simulink model "udp_simulink_example"  (R2022b)
settings: Solver=VariableStepAuto  StartTime=0.0  StopTime=10.0  RelTol=1e-3
libraries: dspnetwork x2
settings Model: Creator=emu  LastModifiedBy=emu

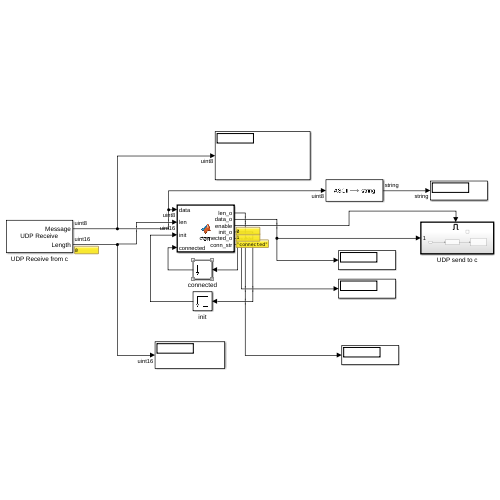
[thumbnail: Simulink's stored preview of the top-level diagram]
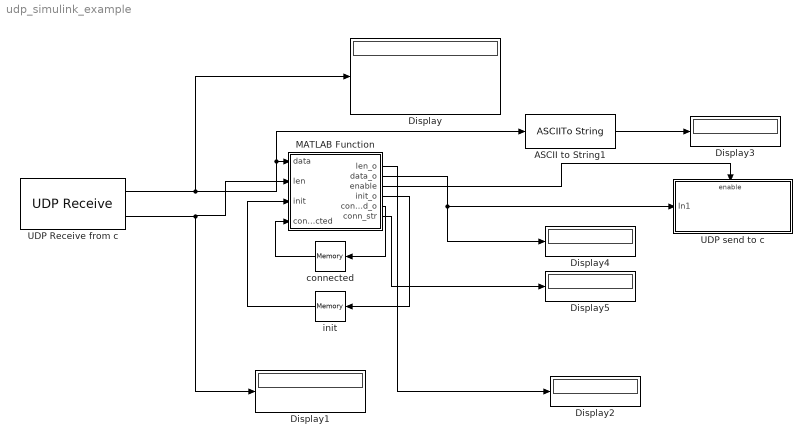
== system udp_simulink_example ==
  ASCII to String1 : ASCIIToString
  Display{,1..5} (6 alike) : Display
  MATLAB Function : MATLAB Function  TreatAsAtomicUnit=on
  UDP Receive from c : dspnetwork/UDP Receive  localURL='0.0.0.0'  localPort=8080  remoteURL='127.0.0.1'  remotePort=-1  recvBufferSize=1024  dims=1024  signalDatatype=uint8  isComplex=off  isVarSize=off  showBlockingTime=off  blockingTime=0  sampletime=1  blockPlatform=[]
      settings: LibrarySourceBlock=dspsrcs4/UDP Receive
  UDP send to c : Subsystem
  connected : Memory
  init : Memory
  wires:
  UDP Receive from c/1 -> ASCII to String1/1, MATLAB Function/1(data), Display/1
  UDP Receive from c/2 -> Display1/1, MATLAB Function/2(len)
  MATLAB Function/1(len_o) -> Display2/1
  connected/1 -> MATLAB Function/4(connected)
  ASCII to String1/1 -> Display3/1
  MATLAB Function/2(data_o) -> Display4/1, UDP send to c/1(In1)
  MATLAB Function/3(enable) -> UDP send to c/Enable
  MATLAB Function/4(init_o) -> init/1
  init/1 -> MATLAB Function/3(init)
  MATLAB Function/5(connected_o) -> connected/1
  MATLAB Function/6(conn_str) -> Display5/1

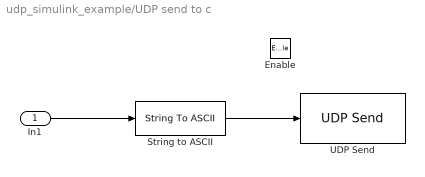
== system udp_simulink_example/UDP send to c ==
  In1 : Inport
  Enable : EnablePort
  String to ASCII : StringToASCII
  UDP Send : dspnetwork/UDP Send  remoteURL='127.0.0.1'  remotePort=8081  localURL='0.0.0.0'  localPortSource=Automatically determine  localPort=8081  sendBufferSize=1024  sampletime=-1  blockPlatform=[]  separateLengthPort=0
      settings: LibrarySourceBlock=dspsnks4/UDP Send
  wires:
  String to ASCII/1 -> UDP Send/1
  In1/1 -> String to ASCII/1

== matlab function udp_simulink_example/MATLAB Function ==
  data: data input; len input; init input; len_o output; connected input; data_o output; enable output; init_o output; connected_o output; conn_str output
function [len_o, data_o, enable, init_o, connected_o, conn_str] = fcn(data, len, init, connected)

len_o = 0;
data_o = "";
enable = 0;
init_o = init;
connected_o = connected;

if(len == 0 && init == 0)
    data_o = "Ist jemand da?";
    enable=1;
    init_o=0;
    len_o = 0;
elseif(len > 0 && init == 0)
    init_o = 1;
end

if(init == 0)
    conn_str = "not connected";
else
    conn_str = "connected";
end

if(len > 0 && init_o == 1)
    len_o = double(len);
    data_o = "Simulink: Habe Daten empfangen!";
    enable = 1;
end
